simulink model "LQR_Practice"  (Simulink 6.0)
settings: Solver=ode45  StartTime=0.0  StopTime=10.0  RelTol=1e-3
values from neighbouring files (symbols this model uses):
  K = lqr(T,Q,Qr,R)    [proj.m]
settings Model: LastModifiedBy=Owner

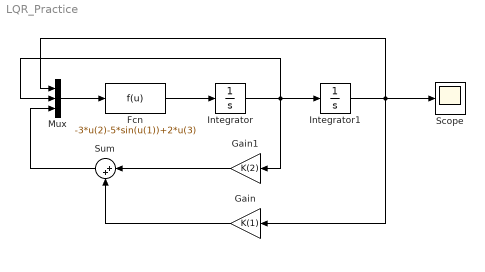
== system LQR_Practice ==
  Fcn : Fcn  Expr=-3*u(2)-5*sin(u(1))+2*u(3)
  Gain : Gain  Orientation=left  Gain=K(1)
  Gain1 : Gain  Orientation=left  Gain=K(2)
  Integrator : Integrator
  Integrator1 : Integrator  InitialCondition=1
  Mux : Mux  Inputs=3
  Scope : Scope
  Sum : Sum  Orientation=left  Inputs=|++
  wires:
  Integrator/1 -> Integrator1/1, Gain1/1, Mux/2
  Integrator1/1 -> Scope/1, Gain/1, Mux/1
  Fcn/1 -> Integrator/1
  Mux/1 -> Fcn/1
  Gain1/1 -> Sum/1
  Gain/1 -> Sum/2
  Sum/1 -> Mux/3
